simulink model "TRN_V2"  (R2020b)
settings: Solver=FixedStepDiscrete  StartTime=0.0  StopTime=300  FixedStep=0.04  RelTol=1e-3
PreLoadFcn:
  | listing = dir;
  | if (contains([listing .name], 'TRN')) && (contains([listing .name], 'MAP'))
  |     addpath('./TRN', './MAP');
  |     addpath( genpath('./MAP') );
  | elseif (contains([listing .name], 'TRN_V2.slx'))
  |     addpath('../TRN', '../MAP');
  |     addpath( genpath('../MAP') );
  | else
  | 
  | end
  | 
  | 
  | load('BusStructureTRNsensor.mat')
settings Model: Creator=wnstj  LastModifiedBy=ASCL
settings OptimizationCC: DefaultParameterBehavior=Inlined  UseDivisionForNetSlopeComputation=on  GainParamInheritBuiltInType=on  UseFloatMulNetSlope=on  InlineInvariantSignals=on  PassReuseOutputArgsAs=Individual arguments  ZeroExternalMemoryAtStartup=off  ZeroInternalMemoryAtStartup=off  NoFixptDivByZeroProtection=on  EfficientFloat2IntCast=on  LifeSpan=1  OptimizeBlockOrder=speed  DifferentSizesBufferReuse=on  EfficientTunableParamExpr=on
settings DebuggingCC: ParameterTunabilityLossMsg=error  SFUnexpectedBacktrackingDiag=warning  SFNoUnconditionalDefaultTransitionDiag=warning  SFMachineParentedDataDiag=error
settings HardwareCC: ProdBitPerPointer=32  ProdBitPerSizeT=32  ProdBitPerPtrDiffT=32  ProdLargestAtomicInteger=Long  ProdLargestAtomicFloat=Double  ProdEndianess=BigEndian  ProdWordSize=32  ProdLongLongMode=on  ProdHWDeviceType=Freescale->MPC83xx
settings ModelReferenceCC: ModelReferenceNumInstancesAllowed=Single
settings SFSimCC: SimUserLibraries=MAPd.lib WS2_32.LIB  MATLABDynamicMemAlloc=off
settings SFSimCC: SimCustomHeaderCode=|
  | #include "MAP.h"
  | #include "MAPDATA.h"
  | #include "DVOF.h"
  | #include "userDefined.h"
settings SFSimCC: SimUserSources=|
  | MAP.c
  | DVOF.c
  | userDefined.c
settings RTWCC: Description=Embedded Coder  SystemTargetFile=ert.tlc  TemplateMakefile=ert_default_tmf  RTWUseSimCustomCode=on  CustomLibrary=MAPd.lib WS2_32.LIB  BuildConfiguration=Debug
settings RTWCC: CustomHeaderCode=|
  | #include "MAP.h"
  | #include "MAPDATA.h"
  | #include "DVOF.h"
  | #include "userDefined.h"
settings RTWCC: CustomSource=|
  | MAP.c
  | DVOF.c
  | userDefined.c
settings CodeAppCC: ForceParamTrailComments=on  IgnoreCustomStorageClasses=off  OperatorAnnotations=on  SimulinkDataObjDesc=on  SFDataObjDesc=on  InsertBlockDesc=on  EnableCustomComments=on
settings ERTTargetCC: TargetLangStandard=C99 (ISO)  GenerateSampleERTMain=on  IncludeMdlTerminateFcn=off  CombineSignalStateStructs=on  SupportAbsoluteTime=off  SupportComplex=off  InlinedParameterPlacement=NonHierarchical  ERTCustomFileTemplate=example_file_process.tlc  ERTFilePackagingFormat=CompactWithDataFile

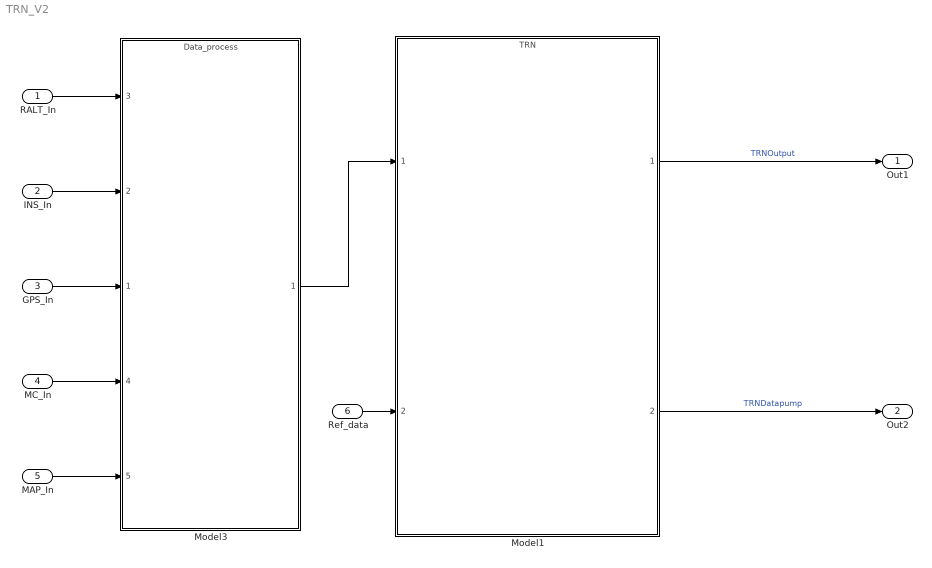
== system TRN_V2 ==
  RALT_In : Inport  OutDataTypeStr=Bus: BUS_SENSOR_RALT  BusOutputAsStruct=on
  INS_In : Inport  Port=2  OutDataTypeStr=Bus: BUS_SENSOR_INS  BusOutputAsStruct=on
  GPS_In : Inport  Port=3  OutDataTypeStr=Bus: BUS_SENSOR_GPS  BusOutputAsStruct=on
  MC_In : Inport  Port=4  OutDataTypeStr=Bus: TRN_MC  BusOutputAsStruct=on
  MAP_In : Inport  Port=5  OutDataTypeStr=Bus: TRN_MAP  BusOutputAsStruct=on
  Ref_data : Inport  Port=6  OutDataTypeStr=Bus: BUS_DYN_STATE  BusOutputAsStruct=on
  Model1 : ModelReference  ModelNameDialog=TRN.slx  SimulationMode=Normal  ModelReferenceVersion=8.261
  Model3 : ModelReference  ModelNameDialog=Data_process.slx  SimulationMode=Normal  ModelReferenceVersion=8.293
      settings: PortSchema="{\"entries\":[{\"content\":{\"sides\":[{\"content\":{\"connectorIds\":[\"In3\",\"In2\",\"In1\",\"In4\",\"In5\"]},\"type\":\"ConnectorPlacement.EquallySpacedRectSide\",\"uuid\":\"f8e947f0-1c4d-433e-a057-358139d8c4fd\"},{\"content\":{\"connectorIds\":[\"Out1\"],\"side\":\"RIGHT\"},\"type\":\"ConnectorPlacement.EquallySpacedRectSide\",\"uuid\":\"9fdbd0a1-e2ed-4384-8f7a-82c9bb56303a\"},{\"content\":{\"connectorIds\":[],\"side\":\"TOP\"},\"type\":\"ConnectorPlacement.EquallySpacedRectSide\",\"uuid\":\"0aae5e4d-7d7d-415a-a081-9af6b9be5f4c\"},{\"content\":{\"connectorIds\":[],\"side\":\"BOTTOM\"},\"type\":\"ConnectorPlacement.EquallySpacedRectSide\",\"uuid\":\"e96609c1-9cad-4ce4-8f73-5a92ad618164\"}]},\"type\":\"ConnectorPlacement.EquallySpacedConnector\",\"uuid\":\"12576536-fd1a-4442-a538-4564d9985bae\"}],\"packageUris\":[\"http://schema.mathworks.com/mf0/Connector/R2020b\"],\"version\":\"1.0\"}"
  Out1 : Outport  OutDataTypeStr=Bus: TRNOutput  VectorParamsAs1DForOutWhenUnconnected=off  BusOutputAsStruct=on
  Out2 : Outport  Port=2  OutDataTypeStr=Bus: TRNDatapump  VectorParamsAs1DForOutWhenUnconnected=off  BusOutputAsStruct=on
  wires:
  Model3/1 -> Model1/1
  RALT_In/1 -> Model3/3
  INS_In/1 -> Model3/2
  GPS_In/1 -> Model3/1
  MC_In/1 -> Model3/4
  MAP_In/1 -> Model3/5
  Model1/2 -> Out2/1  "TRNDatapump"
  Model1/1 -> Out1/1  "TRNOutput"
  Ref_data/1 -> Model1/2
